simulink model "zermelo2b"  (R2017b)
settings: Solver=ode4  StartTime=0.0  StopTime=1  FixedStep=0.02  RelTol=1e-3  EnableMultiTasking=on
values from neighbouring files (symbols this model uses):
  tFinal = thetaFinal(end)    [zermeloMain.m]
  x0 = 4.9    [zermeloMain.m]
  y0 = 1.66    [zermeloMain.m]
settings Model: Creator=Soutrik  LastModifiedBy=Soutrik

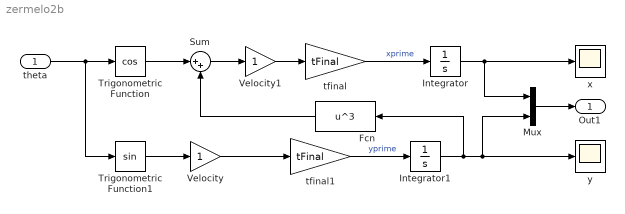
== system zermelo2b ==
  theta : Inport
  Fcn : Fcn  Expr=u^3
  Integrator : Integrator  InitialCondition=x0
  Integrator1 : Integrator  InitialCondition=y0
  Mux : Mux  Inputs=2
  Sum : Sum  Inputs=|++
  Trigonometric Function : Trigonometry  Operator=cos
  Trigonometric Function1 : Trigonometry
  Velocity : Gain
  Velocity1 : Gain
  tfinal : Gain  Gain=tFinal
  tfinal1 : Gain  Gain=tFinal
  x : Scope
  y : Scope
  Out1 : Outport
  wires:
  Velocity1/1 -> tfinal/1
  tfinal/1 -> Integrator/1  "xprime"
  Trigonometric Function/1 -> Sum/1
  Integrator/1 -> Mux/1, x/1
  tfinal1/1 -> Integrator1/1  "yprime"
  Mux/1 -> Out1/1
  Integrator1/1 -> Fcn/1, Mux/2, y/1
  Trigonometric Function1/1 -> Velocity/1
  Sum/1 -> Velocity1/1
  theta/1 -> Trigonometric Function1/1, Trigonometric Function/1
  Velocity/1 -> tfinal1/1
  Fcn/1 -> Sum/2
